simulink model "nav_flocking4"  (R2022b)
settings: Solver=FixedStepAuto  StartTime=0.0  StopTime=10.0  FixedStep=0.01  RelTol=1e-3
values from neighbouring files (symbols this model uses):
  a = 1    [main_flock3.m]    (also in main_flock4.m; params_flocking_ros.m)
  aR = diag([ar; ap; ay])    [main_flock3.m]    (also in main_flock4.m; main_sliding.m)
  Att1 = [2 -2 -15]    [main_flock3.m]    (also in main_flock4.m)
  Att2 = [2 -2 -15]    [main_flock3.m]    (also in main_flock4.m)
  Att3 = [2 -2 -15]    [main_flock3.m]    (also in main_flock4.m)
  Att4 = [2 -2 -15]    [main_flock4.m]
  b = 1    [main_flock3.m]    (also in main_flock4.m; params_flocking_ros.m)
  c = 1    [main_flock3.m]    (also in main_flock4.m; params_flocking_ros.m)
  c_gammap = 1.2    [main_flock3.m]    (also in main_flock4.m)
  c_gammav = 3.5    [main_flock3.m]    (also in main_flock4.m)
  d = 0.6    [main_flock3.m]    (also in main_flock4.m; params_flocking_ros.m)
  d_prime = 1    [main_flock3.m]    (also in main_flock4.m; params_flocking_ros.m)
  epsilon = 0.1    [main_flock3.m]    (also in main_flock4.m; params_flocking_ros.m)
  h = 0.2    [main_flock3.m]    (also in main_flock4.m; params_flocking_ros.m)
  K1 = diag([k111; k122; k133])    [main_flock3.m]    (also in main_flock4.m; main_sliding.m)
  K2 = diag([k211; k222; k233])    [main_flock3.m]    (also in main_flock4.m; main_sliding.m)
  Ki = diag([Ki1; Ki2; Ki3])    [main_flock3.m]    (also in main_flock4.m; main_sliding.m)
  lam = diag([lam1; lam2; lam3])    [main_flock3.m]    (also in main_flock4.m; main_sliding.m)
  R = 0.15    [main_flock3.m]    (also in main_flock4.m; params_flocking_ros.m)
  vxobs = 0    [main_flock3.m]    (also in main_flock4.m)
  vyobs = 0    [main_flock3.m]    (also in main_flock4.m)
  vzobs = 0    [main_flock3.m]    (also in main_flock4.m)
  X0_1 = [P01 dP01 om01]    [main_flock3.m]    (also in main_flock4.m; main_sliding.m = [P0 dP0 om0])
  X0_2 = [P02 dP02 om02]    [main_flock3.m]    (also in main_flock4.m)
  X0_3 = [P03 dP03 om03]    [main_flock3.m]    (also in main_flock4.m)
  X0_4 = [P04 dP04 om04]    [main_flock4.m]
  xmax = 2    [main_flock3.m]    (also in main_flock4.m)
  xmin = -2    [main_flock3.m]    (also in main_flock4.m)
  xobs = 0.75    [main_flock3.m]    (also in main_flock4.m)
  yobs = -0.25    [main_flock3.m]    (also in main_flock4.m)
  zobs = 1.7    [main_flock3.m]    (also in main_flock4.m)
undefined symbols (not defined in the file or in its folder): A_Euler
libraries: aerosimlib x4
(part 1 of 3)
settings Model: Creator=root  LastModifiedBy=jonatan_alvarez
settings SolverCC: AlgebraicLoopSolver=TrustRegion
settings DataIOCC: ReturnWorkspaceOutputs=off
settings DebuggingCC: UnconnectedInputMsg=warning  UnconnectedOutputMsg=warning  UnconnectedLineMsg=warning  SFMachineParentedDataDiag=warning  UnderSpecifiedDimensionMsg=warning  ArithmeticOperatorsInVariantConditions=warning
settings ModelReferenceCC: EnableRefExpFcnMdlSchedulingChecks=on
settings SFSimCC: CustomCodeUndefinedFunction=UseInterfaceOnly

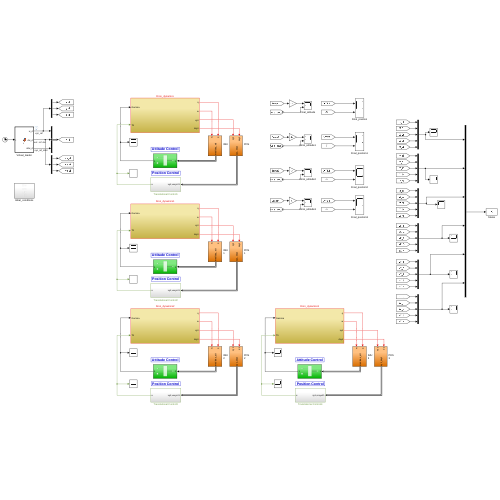
[thumbnail: Simulink's stored preview of the top-level diagram]
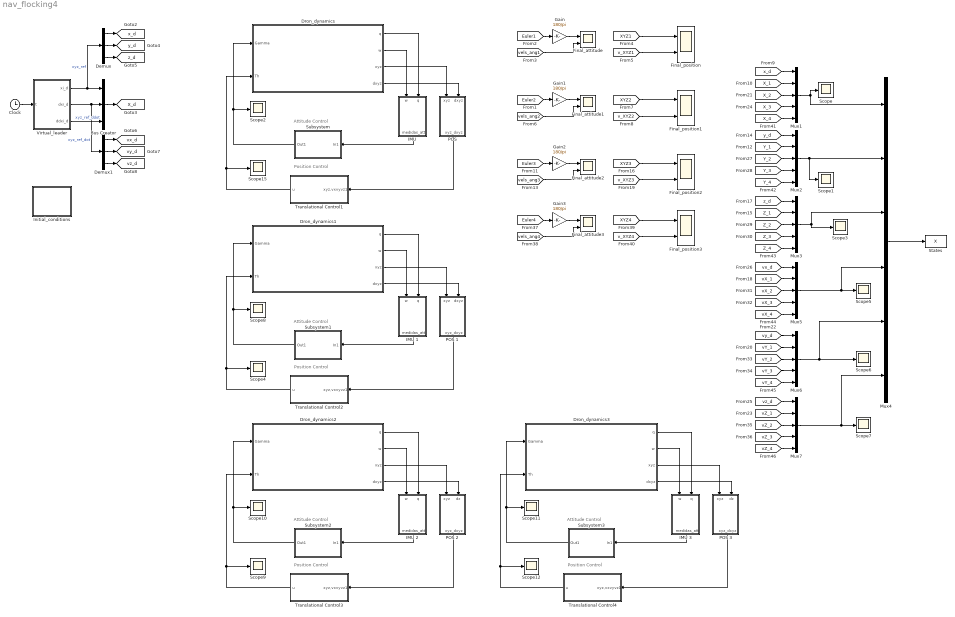
== system nav_flocking4 ==
  note: Position Control
  note: Attitude Control
  note: Position Control
  note: Attitude Control
  note: Position Control
  note: Attitude Control
  note: Position Control
  note: Attitude Control
  Bus Creator : BusCreator  Inputs=3
  Clock : Clock
  Demux : Demux  Outputs=3
  Demux1 : Demux  Outputs=3
  Dron_dynamics : Subsystem
  Dron_dynamics1 : Subsystem
  Dron_dynamics2 : Subsystem
  Dron_dynamics3 : Subsystem
  Final_attitude{,1..3} (4 alike) : Scope  NumInputPorts=2
  Final_position{,1..3} (4 alike) : Scope  NumInputPorts=2
  Gain{,1..3} (4 alike) : Gain  Gain=180/pi
  "IMU " : Subsystem
  IMU 1 : Subsystem
  IMU 2 : Subsystem
  IMU 3 : Subsystem
  Initial_conditions : Subsystem
  Mux{1..3,5..7} (6 alike) : Mux  Inputs=5
  Mux4 : Mux  Inputs=6
  "POS " : Subsystem
  POS 1 : Subsystem
  POS 2 : Subsystem
  POS 3 : Subsystem
  Scope{,1..12,15} (14 alike) : Scope
  States : ToWorkspace  VariableName=X  SampleTime=-1
  Subsystem : Subsystem
  Subsystem1 : Subsystem
  Subsystem2 : Subsystem
  Subsystem3 : Subsystem
  Translational Control1 : Subsystem
  Translational Control2 : Subsystem
  Translational Control3 : Subsystem
  Translational Control4 : Subsystem
  Virtual_leader : MATLAB Function  TreatAsAtomicUnit=on
  tag scope: X_d=global, vx_d=global, vy_d=global, vz_d=global, x_d=global, y_d=global, z_d=global
  wires:
  [vels_ang1] -> Final_attitude/2
  [v_XYZ1] -> Final_position/2
  Gain/1 -> Final_attitude/1
  [XYZ1] -> Final_position/1
  [Euler1] -> Gain/1
  Dron_dynamics/2(w) -> "IMU "/1(w)
  Dron_dynamics/4(dxyz) -> "POS "/2(dxyz)
  Bus Creator/1 -> [X_d]
  Virtual_leader/3(ddxi_d) -> Bus Creator/3  "xyz_ref_ddot"
  Dron_dynamics/1(q) -> "IMU "/2(q)
  Subsystem/1(Out1) -> Scope2/1, Dron_dynamics/1(Gamma)
  Dron_dynamics/3(xyz) -> "POS "/1(xyz)
  "POS "/1(xyz_dxyz) -> Translational Control1/1(xyz,vxvyvz1)
  Translational Control1/1(u) -> Scope15/1, Dron_dynamics/2(Th)
  "IMU "/1(medidas_att) -> Subsystem/1(In1)
  Virtual_leader/1(xi_d) -> Demux/1, Bus Creator/1  "xyz_ref"
  Demux/1 -> [x_d]
  Demux/2 -> [y_d]
  Demux/3 -> [z_d]
  [x_d] -> Mux1/1
  [X_1] -> Mux1/2
  Mux2/1 -> Scope1/1, Mux4/2
  [Y_1] -> Mux2/2
  [y_d] -> Mux2/1
  [z_d] -> Mux3/1
  [Z_1] -> Mux3/2
  Mux3/1 -> Mux4/3, Scope3/1
  Mux4/1 -> States/1
  Mux1/1 -> Scope/1, Mux4/1
  Demux1/3 -> [vz_d]
  Demux1/2 -> [vy_d]
  Demux1/1 -> [vx_d]
  Virtual_leader/2(dxi_d) -> Demux1/1, Bus Creator/2  "xyz_ref_dot"
  [vZ_1] -> Mux7/2
  [vz_d] -> Mux7/1
  [vy_d] -> Mux6/1
  [vY_1] -> Mux6/2
  [vX_1] -> Mux5/2
  [vx_d] -> Mux5/1
  Mux5/1 -> Mux4/4, Scope5/1
  Mux6/1 -> Mux4/5, Scope6/1
  Mux7/1 -> Mux4/6, Scope7/1
  Clock/1 -> Virtual_leader/1(t)
  Dron_dynamics1/2(w) -> IMU 1/1(w)
  Dron_dynamics1/4(dxyz) -> POS 1/2(dxyz)
  Dron_dynamics1/3(xyz) -> POS 1/1(xyz)
  POS 1/1(xyz_dxyz) -> Translational Control2/1(xyz,vxvyvz1)
  Dron_dynamics1/1(q) -> IMU 1/2(q)
  Translational Control2/1(u) -> Scope4/1, Dron_dynamics1/2(Th)
  IMU 1/1(medidas_att) -> Subsystem1/1(In1)
  Subsystem1/1(Out1) -> Scope8/1, Dron_dynamics1/1(Gamma)
  Dron_dynamics2/2(w) -> IMU 2/1(w)
  Dron_dynamics2/4(dxyz) -> POS 2/2(dz)
  Dron_dynamics2/3(xyz) -> POS 2/1(xyz)
  POS 2/1(xyz_dxyz) -> Translational Control3/1(xyz,vxvyvz1)
  Dron_dynamics2/1(q) -> IMU 2/2(q)
  Translational Control3/1(u) -> Scope9/1, Dron_dynamics2/2(Th)
  IMU 2/1(medidas_att) -> Subsystem2/1(In1)
  Subsystem2/1(Out1) -> Scope10/1, Dron_dynamics2/1(Gamma)
  [v_XYZ2] -> Final_position1/2
  [Euler2] -> Gain1/1
  Gain1/1 -> Final_attitude1/1
  [XYZ2] -> Final_position1/1
  [vels_ang2] -> Final_attitude1/2
  [v_XYZ3] -> Final_position2/2
  [Euler3] -> Gain2/1
  Gain2/1 -> Final_attitude2/1
  [XYZ3] -> Final_position2/1
  [vels_ang3] -> Final_attitude2/2
  [X_2] -> Mux1/3
  [X_3] -> Mux1/4
  [Y_2] -> Mux2/3
  [Y_3] -> Mux2/4
  [Z_2] -> Mux3/3
  [Z_3] -> Mux3/4
  [vX_2] -> Mux5/3
  [vX_3] -> Mux5/4
  [vY_2] -> Mux6/3
  [vY_3] -> Mux6/4
  [vZ_2] -> Mux7/3
  [vZ_3] -> Mux7/4
  Subsystem3/1(Out1) -> Dron_dynamics3/1(Gamma), Scope11/1
  IMU 3/1(medidas_att) -> Subsystem3/1(In1)
  Translational Control4/1(u) -> Dron_dynamics3/2(Th), Scope12/1
  Dron_dynamics3/1(q) -> IMU 3/2(q)
  POS 3/1(xyz_dxyz) -> Translational Control4/1(xyz,vxvyvz1)
  Dron_dynamics3/3(xyz) -> POS 3/1(xyz)
  Dron_dynamics3/4(dxyz) -> POS 3/2(dz)
  Dron_dynamics3/2(w) -> IMU 3/1(w)
  [vels_ang4] -> Final_attitude3/2
  [XYZ4] -> Final_position3/1
  Gain3/1 -> Final_attitude3/1
  [Euler4] -> Gain3/1
  [v_XYZ4] -> Final_position3/2
  [X_4] -> Mux1/5
  [Y_4] -> Mux2/5
  [Z_4] -> Mux3/5
  [vX_4] -> Mux5/5
  [vY_4] -> Mux6/5
  [vZ_4] -> Mux7/5

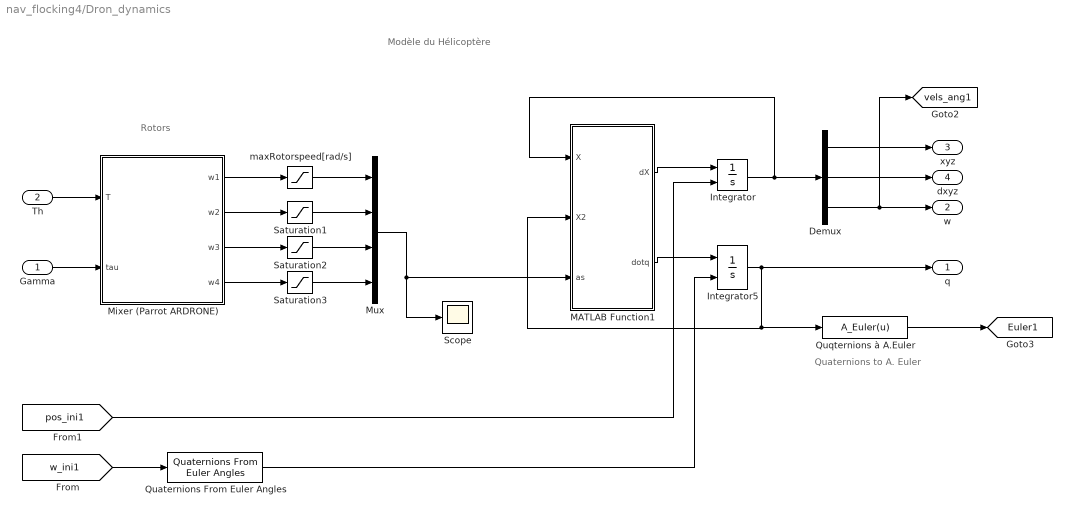
== system nav_flocking4/Dron_dynamics ==
  note: Modèle du Hélicoptère
  note: Rotors
  note: Quaternions to A. Euler
  Gamma : Inport
  Th : Inport  Port=2
  Demux : Demux  Outputs=3
  Integrator : Integrator  InitialConditionSource=external
  Integrator5 : Integrator  InitialConditionSource=external  InitialCondition=[1 0 0 0]
  MATLAB Function1 : MATLAB Function  TreatAsAtomicUnit=on
  Mixer (Parrot ARDRONE) : MATLAB Function  TreatAsAtomicUnit=on
  Mux : Mux
  Quaternions From Euler Angles : aerosimlib/Transformations/Quaternions From Euler Angles
  Quqternions à A.Euler : MATLABFcn  MATLABFcn=A_Euler(u)  OutputDimensions=3
  Saturation1 : Saturate  UpperLimit=1100  LowerLimit=5
  Saturation2 : Saturate  UpperLimit=1100  LowerLimit=5
  Saturation3 : Saturate  UpperLimit=1100  LowerLimit=5
  Scope : Scope
  maxRotorspeed[rad/s] : Saturate  UpperLimit=1100  LowerLimit=5
  q : Outport  VectorParamsAs1DForOutWhenUnconnected=off
  w : Outport  Port=2  VectorParamsAs1DForOutWhenUnconnected=off
  xyz : Outport  Port=3  VectorParamsAs1DForOutWhenUnconnected=off
  dxyz : Outport  Port=4  VectorParamsAs1DForOutWhenUnconnected=off
  tag scope: Euler1=global, vels_ang1=global
  wires:
  [w_ini1] -> Quaternions From Euler Angles/1
  Quqternions à A.Euler/1 -> [Euler1]
  Mixer (Parrot ARDRONE)/4(w4) -> Saturation3/1
  Saturation1/1 -> Mux/2
  Mixer (Parrot ARDRONE)/2(w2) -> Saturation1/1
  Mixer (Parrot ARDRONE)/1(w1) -> maxRotorspeed[rad/s]/1
  maxRotorspeed[rad/s]/1 -> Mux/1
  Saturation3/1 -> Mux/4
  Saturation2/1 -> Mux/3
  Mixer (Parrot ARDRONE)/3(w3) -> Saturation2/1
  Mux/1 -> Scope/1, MATLAB Function1/3(as)
  Integrator5/1 -> MATLAB Function1/2(X2), Quqternions à A.Euler/1, q/1
  MATLAB Function1/1(dX) -> Integrator/1
  MATLAB Function1/2(dotq) -> Integrator5/1
  Quaternions From Euler Angles/1 -> Integrator5/2
  Integrator/1 -> Demux/1, MATLAB Function1/1(X)
  Gamma/1 -> Mixer (Parrot ARDRONE)/2(tau)
  [pos_ini1] -> Integrator/2
  Demux/3 -> [vels_ang1], w/1
  Demux/1 -> xyz/1
  Demux/2 -> dxyz/1
  Th/1 -> Mixer (Parrot ARDRONE)/1(T)

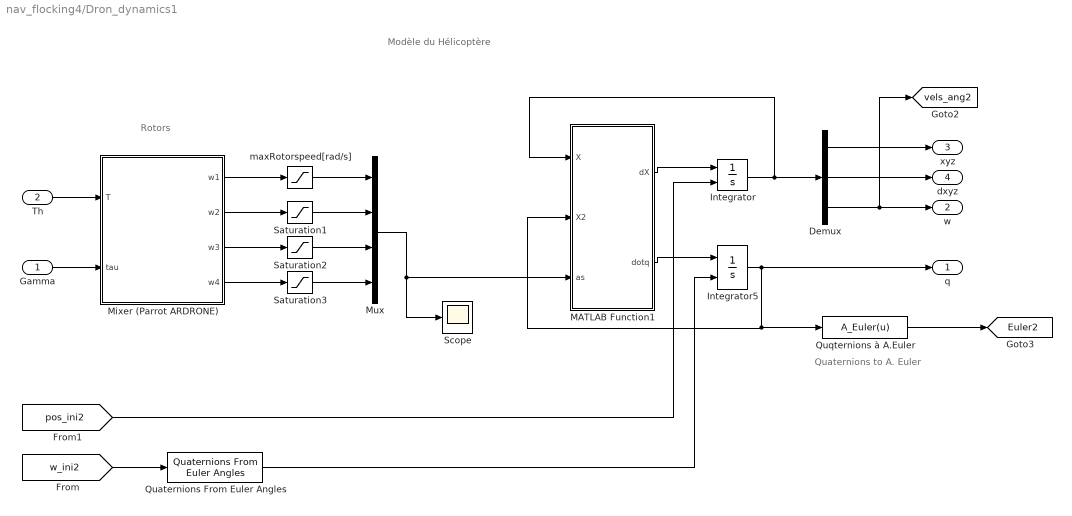
== system nav_flocking4/Dron_dynamics1 ==
  note: Modèle du Hélicoptère
  note: Rotors
  note: Quaternions to A. Euler
  Gamma : Inport
  Th : Inport  Port=2
  Demux : Demux  Outputs=3
  Integrator : Integrator  InitialConditionSource=external
  Integrator5 : Integrator  InitialConditionSource=external  InitialCondition=[1 0 0 0]
  MATLAB Function1 : MATLAB Function  TreatAsAtomicUnit=on
  Mixer (Parrot ARDRONE) : MATLAB Function  TreatAsAtomicUnit=on
  Mux : Mux
  Quaternions From Euler Angles : aerosimlib/Transformations/Quaternions From Euler Angles
  Quqternions à A.Euler : MATLABFcn  MATLABFcn=A_Euler(u)  OutputDimensions=3
  Saturation1 : Saturate  UpperLimit=1100  LowerLimit=5
  Saturation2 : Saturate  UpperLimit=1100  LowerLimit=5
  Saturation3 : Saturate  UpperLimit=1100  LowerLimit=5
  Scope : Scope
  maxRotorspeed[rad/s] : Saturate  UpperLimit=1100  LowerLimit=5
  q : Outport  VectorParamsAs1DForOutWhenUnconnected=off
  w : Outport  Port=2  VectorParamsAs1DForOutWhenUnconnected=off
  xyz : Outport  Port=3  VectorParamsAs1DForOutWhenUnconnected=off
  dxyz : Outport  Port=4  VectorParamsAs1DForOutWhenUnconnected=off
  tag scope: Euler2=global, vels_ang2=global
  wires:
  [w_ini2] -> Quaternions From Euler Angles/1
  Quqternions à A.Euler/1 -> [Euler2]
  Mixer (Parrot ARDRONE)/4(w4) -> Saturation3/1
  Saturation1/1 -> Mux/2
  Mixer (Parrot ARDRONE)/2(w2) -> Saturation1/1
  Mixer (Parrot ARDRONE)/1(w1) -> maxRotorspeed[rad/s]/1
  maxRotorspeed[rad/s]/1 -> Mux/1
  Saturation3/1 -> Mux/4
  Saturation2/1 -> Mux/3
  Mixer (Parrot ARDRONE)/3(w3) -> Saturation2/1
  Mux/1 -> Scope/1, MATLAB Function1/3(as)
  Integrator5/1 -> MATLAB Function1/2(X2), Quqternions à A.Euler/1, q/1
  MATLAB Function1/1(dX) -> Integrator/1
  MATLAB Function1/2(dotq) -> Integrator5/1
  Quaternions From Euler Angles/1 -> Integrator5/2
  Integrator/1 -> Demux/1, MATLAB Function1/1(X)
  Gamma/1 -> Mixer (Parrot ARDRONE)/2(tau)
  [pos_ini2] -> Integrator/2
  Demux/3 -> [vels_ang2], w/1
  Demux/1 -> xyz/1
  Demux/2 -> dxyz/1
  Th/1 -> Mixer (Parrot ARDRONE)/1(T)

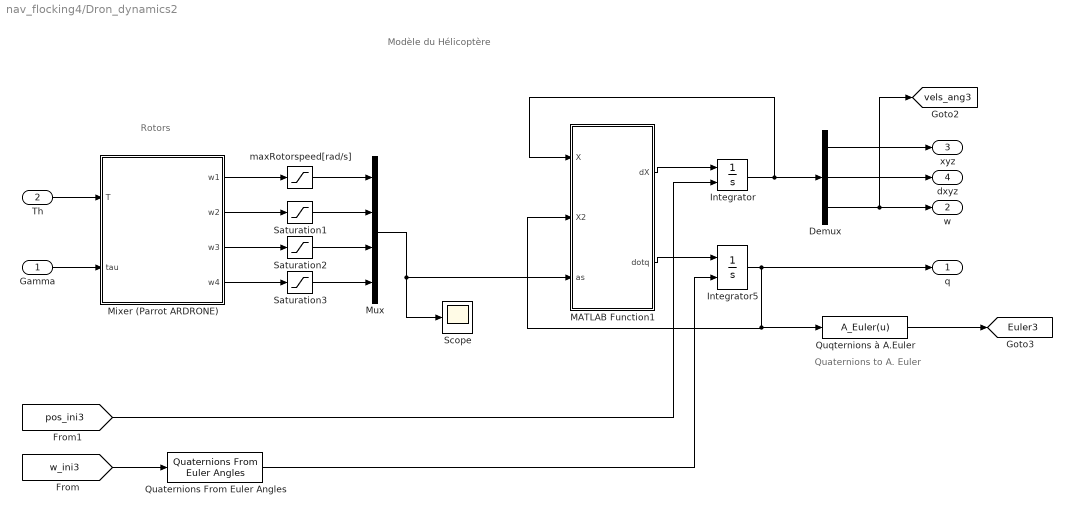
== system nav_flocking4/Dron_dynamics2 ==
  note: Modèle du Hélicoptère
  note: Rotors
  note: Quaternions to A. Euler
  Gamma : Inport
  Th : Inport  Port=2
  Demux : Demux  Outputs=3
  Integrator : Integrator  InitialConditionSource=external
  Integrator5 : Integrator  InitialConditionSource=external  InitialCondition=[1 0 0 0]
  MATLAB Function1 : MATLAB Function  TreatAsAtomicUnit=on
  Mixer (Parrot ARDRONE) : MATLAB Function  TreatAsAtomicUnit=on
  Mux : Mux
  Quaternions From Euler Angles : aerosimlib/Transformations/Quaternions From Euler Angles
  Quqternions à A.Euler : MATLABFcn  MATLABFcn=A_Euler(u)  OutputDimensions=3
  Saturation1 : Saturate  UpperLimit=1100  LowerLimit=5
  Saturation2 : Saturate  UpperLimit=1100  LowerLimit=5
  Saturation3 : Saturate  UpperLimit=1100  LowerLimit=5
  Scope : Scope
  maxRotorspeed[rad/s] : Saturate  UpperLimit=1100  LowerLimit=5
  q : Outport  VectorParamsAs1DForOutWhenUnconnected=off
  w : Outport  Port=2  VectorParamsAs1DForOutWhenUnconnected=off
  xyz : Outport  Port=3  VectorParamsAs1DForOutWhenUnconnected=off
  dxyz : Outport  Port=4  VectorParamsAs1DForOutWhenUnconnected=off
  tag scope: Euler3=global, vels_ang3=global
  wires:
  [w_ini3] -> Quaternions From Euler Angles/1
  Quqternions à A.Euler/1 -> [Euler3]
  Mixer (Parrot ARDRONE)/4(w4) -> Saturation3/1
  Saturation1/1 -> Mux/2
  Mixer (Parrot ARDRONE)/2(w2) -> Saturation1/1
  Mixer (Parrot ARDRONE)/1(w1) -> maxRotorspeed[rad/s]/1
  maxRotorspeed[rad/s]/1 -> Mux/1
  Saturation3/1 -> Mux/4
  Saturation2/1 -> Mux/3
  Mixer (Parrot ARDRONE)/3(w3) -> Saturation2/1
  Mux/1 -> Scope/1, MATLAB Function1/3(as)
  Integrator5/1 -> MATLAB Function1/2(X2), Quqternions à A.Euler/1, q/1
  MATLAB Function1/1(dX) -> Integrator/1
  MATLAB Function1/2(dotq) -> Integrator5/1
  Quaternions From Euler Angles/1 -> Integrator5/2
  Integrator/1 -> Demux/1, MATLAB Function1/1(X)
  Gamma/1 -> Mixer (Parrot ARDRONE)/2(tau)
  [pos_ini3] -> Integrator/2
  Demux/3 -> [vels_ang3], w/1
  Demux/1 -> xyz/1
  Demux/2 -> dxyz/1
  Th/1 -> Mixer (Parrot ARDRONE)/1(T)

== system nav_flocking4/Dron_dynamics3 ==
  note: Quaternions to A. Euler
  note: Rotors
  note: Modèle du Hélicoptère
  Gamma : Inport
  Th : Inport  Port=2
  Demux : Demux  Outputs=3
  Integrator : Integrator  InitialConditionSource=external
  Integrator5 : Integrator  InitialConditionSource=external  InitialCondition=[1 0 0 0]
  MATLAB Function1 : MATLAB Function  TreatAsAtomicUnit=on
  Mixer (Parrot ARDRONE) : MATLAB Function  TreatAsAtomicUnit=on
  Mux : Mux
  Quaternions From Euler Angles : aerosimlib/Transformations/Quaternions From Euler Angles
  Quqternions à A.Euler : MATLABFcn  MATLABFcn=A_Euler(u)  OutputDimensions=3
  Saturation1 : Saturate  UpperLimit=1100  LowerLimit=5
  Saturation2 : Saturate  UpperLimit=1100  LowerLimit=5
  Saturation3 : Saturate  UpperLimit=1100  LowerLimit=5
  Scope : Scope
  maxRotorspeed[rad/s] : Saturate  UpperLimit=1100  LowerLimit=5
  q : Outport  VectorParamsAs1DForOutWhenUnconnected=off
  w : Outport  Port=2  VectorParamsAs1DForOutWhenUnconnected=off
  xyz : Outport  Port=3  VectorParamsAs1DForOutWhenUnconnected=off
  dxyz : Outport  Port=4  VectorParamsAs1DForOutWhenUnconnected=off
  tag scope: Euler4=global, vels_ang4=global
  wires:
  Th/1 -> Mixer (Parrot ARDRONE)/1(T)
  Demux/2 -> dxyz/1
  Demux/1 -> xyz/1
  Demux/3 -> w/1, [vels_ang4]
  [pos_ini4] -> Integrator/2
  Gamma/1 -> Mixer (Parrot ARDRONE)/2(tau)
  Integrator/1 -> MATLAB Function1/1(X), Demux/1
  Quaternions From Euler Angles/1 -> Integrator5/2
  MATLAB Function1/2(dotq) -> Integrator5/1
  MATLAB Function1/1(dX) -> Integrator/1
  Integrator5/1 -> q/1, Quqternions à A.Euler/1, MATLAB Function1/2(X2)
  Mux/1 -> MATLAB Function1/3(as), Scope/1
  Mixer (Parrot ARDRONE)/3(w3) -> Saturation2/1
  Saturation2/1 -> Mux/3
  Saturation3/1 -> Mux/4
  maxRotorspeed[rad/s]/1 -> Mux/1
  Mixer (Parrot ARDRONE)/1(w1) -> maxRotorspeed[rad/s]/1
  Mixer (Parrot ARDRONE)/2(w2) -> Saturation1/1
  Saturation1/1 -> Mux/2
  Mixer (Parrot ARDRONE)/4(w4) -> Saturation3/1
  Quqternions à A.Euler/1 -> [Euler4]
  [w_ini4] -> Quaternions From Euler Angles/1

== system nav_flocking4/IMU  ==
  w : Inport
  q : Inport  Port=2
  Bus Creator : BusCreator  Inputs=4
  Display : Display
  Integrator : Integrator
  Scope : Scope
  q_e : Subsystem
  medidas_att : Outport  VectorParamsAs1DForOutWhenUnconnected=off
  wires:
  [q_d1] -> q_e/1(q1)
  q/1 -> Bus Creator/1, q_e/2(Q2)
  w/1 -> Bus Creator/3
  Integrator/1 -> Display/1, Bus Creator/4
  Bus Creator/1 -> medidas_att/1
  q_e/1(qxQ) -> Integrator/1, Scope/1, Bus Creator/2

== system nav_flocking4/IMU 1 ==
  w : Inport
  q : Inport  Port=2
  Bus Creator : BusCreator  Inputs=4
  Display : Display
  Integrator : Integrator
  Scope : Scope
  q_e : Subsystem
  medidas_att : Outport  VectorParamsAs1DForOutWhenUnconnected=off
  wires:
  [q_d2] -> q_e/1(q1)
  q/1 -> Bus Creator/1, q_e/2(Q2)
  w/1 -> Bus Creator/3
  Integrator/1 -> Display/1, Bus Creator/4
  Bus Creator/1 -> medidas_att/1
  q_e/1(qxQ) -> Integrator/1, Scope/1, Bus Creator/2

== system nav_flocking4/IMU 2 ==
  w : Inport
  q : Inport  Port=2
  Bus Creator : BusCreator  Inputs=4
  Display : Display
  Integrator : Integrator
  Scope : Scope
  q_e : Subsystem
  medidas_att : Outport  VectorParamsAs1DForOutWhenUnconnected=off
  wires:
  [q_d3] -> q_e/1(q1)
  q/1 -> Bus Creator/1, q_e/2(Q2)
  w/1 -> Bus Creator/3
  Integrator/1 -> Display/1, Bus Creator/4
  Bus Creator/1 -> medidas_att/1
  q_e/1(qxQ) -> Integrator/1, Scope/1, Bus Creator/2

== system nav_flocking4/IMU 3 ==
  w : Inport
  q : Inport  Port=2
  Bus Creator : BusCreator  Inputs=4
  Display : Display
  Integrator : Integrator
  Scope : Scope
  q_e : Subsystem
  medidas_att : Outport  VectorParamsAs1DForOutWhenUnconnected=off
  wires:
  q_e/1(qxQ) -> Bus Creator/2, Scope/1, Integrator/1
  Bus Creator/1 -> medidas_att/1
  Integrator/1 -> Bus Creator/4, Display/1
  w/1 -> Bus Creator/3
  q/1 -> q_e/2(Q2), Bus Creator/1
  [q_d4] -> q_e/1(q1)

== system nav_flocking4/Initial_conditions ==
  "phi, theta,psi Condition Initiale" : Constant  Value=[Att1]*pi/180
  "phi, theta,psi Condition Initiale1" : Constant  Value=X0_1
  "phi, theta,psi Condition Initiale2" : Constant  Value=[Att2]*pi/180
  "phi, theta,psi Condition Initiale3" : Constant  Value=X0_2
  "phi, theta,psi Condition Initiale4" : Constant  Value=[Att3]*pi/180
  "phi, theta,psi Condition Initiale5" : Constant  Value=X0_3
  "phi, theta,psi Condition Initiale6" : Constant  Value=[Att4]*pi/180
  "phi, theta,psi Condition Initiale7" : Constant  Value=X0_4
  tag scope: pos_ini1=global, pos_ini2=global, pos_ini3=global, pos_ini4=global, w_ini1=global, w_ini2=global, w_ini3=global, w_ini4=global
  wires:
  "phi, theta,psi Condition Initiale1"/1 -> [pos_ini1]
  "phi, theta,psi Condition Initiale"/1 -> [w_ini1]
  "phi, theta,psi Condition Initiale2"/1 -> [w_ini2]
  "phi, theta,psi Condition Initiale3"/1 -> [pos_ini2]
  "phi, theta,psi Condition Initiale4"/1 -> [w_ini3]
  "phi, theta,psi Condition Initiale5"/1 -> [pos_ini3]
  "phi, theta,psi Condition Initiale7"/1 -> [pos_ini4]
  "phi, theta,psi Condition Initiale6"/1 -> [w_ini4]

== system nav_flocking4/POS  ==
  xyz : Inport
  dxyz : Inport  Port=2
  Bus Creator : BusCreator  Inputs=2
  Demux : Demux  Outputs=3
  Demux1 : Demux  Outputs=3
  States : ToWorkspace  VariableName=X1  SampleTime=-1
  xyz_dxyz : Outport  VectorParamsAs1DForOutWhenUnconnected=off
  tag scope: XYZ1=global, X_1=global, Y_1=global, Z_1=global, states1=global, vX_1=global, vY_1=global, vZ_1=global, v_XYZ1=global
  wires:
  xyz/1 -> Bus Creator/1, States/1, Demux/1, [XYZ1]  "xyz"
  dxyz/1 -> Bus Creator/2, Demux1/1, [v_XYZ1]  "xyz_dot"
  Demux/1 -> [X_1]
  Demux/2 -> [Y_1]
  Demux/3 -> [Z_1]
  Demux1/3 -> [vZ_1]
  Demux1/2 -> [vY_1]
  Demux1/1 -> [vX_1]
  Bus Creator/1 -> [states1], xyz_dxyz/1

== system nav_flocking4/POS 1 ==
  xyz : Inport
  dxyz : Inport  Port=2
  Bus Creator : BusCreator  Inputs=2
  Demux : Demux  Outputs=3
  Demux1 : Demux  Outputs=3
  States : ToWorkspace  VariableName=X2  SampleTime=-1
  xyz_dxyz : Outport  VectorParamsAs1DForOutWhenUnconnected=off
  tag scope: XYZ2=global, X_2=global, Y_2=global, Z_2=global, states2=global, vX_2=global, vY_2=global, vZ_2=global, v_XYZ2=global
  wires:
  xyz/1 -> Bus Creator/1, States/1, Demux/1, [XYZ2]  "xyz"
  dxyz/1 -> Bus Creator/2, Demux1/1, [v_XYZ2]  "xyz_dot"
  Demux/1 -> [X_2]
  Demux/2 -> [Y_2]
  Demux/3 -> [Z_2]
  Bus Creator/1 -> [states2], xyz_dxyz/1
  Demux1/3 -> [vZ_2]
  Demux1/2 -> [vY_2]
  Demux1/1 -> [vX_2]

== system nav_flocking4/POS 2 ==
  xyz : Inport
  dz : Inport  Port=2
  Bus Creator : BusCreator  Inputs=2
  Demux : Demux  Outputs=3
  Demux1 : Demux  Outputs=3
  States : ToWorkspace  VariableName=X3  SampleTime=-1
  xyz_dxyz : Outport  VectorParamsAs1DForOutWhenUnconnected=off
  tag scope: XYZ3=global, X_3=global, Y_3=global, Z_3=global, states3=global, vX_3=global, vY_3=global, vZ_3=global, v_XYZ3=global
  wires:
  xyz/1 -> Bus Creator/1, States/1, Demux/1, [XYZ3]  "xyz"
  dz/1 -> Bus Creator/2, Demux1/1, [v_XYZ3]  "xyz_dot"
  Demux/1 -> [X_3]
  Demux/2 -> [Y_3]
  Demux/3 -> [Z_3]
  Bus Creator/1 -> [states3], xyz_dxyz/1
  Demux1/3 -> [vZ_3]
  Demux1/2 -> [vY_3]
  Demux1/1 -> [vX_3]

== system nav_flocking4/POS 3 ==
  xyz : Inport
  dz : Inport  Port=2
  Bus Creator : BusCreator  Inputs=2
  Demux : Demux  Outputs=3
  Demux1 : Demux  Outputs=3
  States : ToWorkspace  VariableName=X4  SampleTime=-1
  xyz_dxyz : Outport  VectorParamsAs1DForOutWhenUnconnected=off
  tag scope: XYZ4=global, X_4=global, Y_4=global, Z_4=global, states4=global, vX_4=global, vY_4=global, vZ_4=global, v_XYZ4=global
  wires:
  Demux1/1 -> [vX_4]
  Demux1/2 -> [vY_4]
  Demux1/3 -> [vZ_4]
  Bus Creator/1 -> xyz_dxyz/1, [states4]
  Demux/3 -> [Z_4]
  Demux/2 -> [Y_4]
  Demux/1 -> [X_4]
  dz/1 -> [v_XYZ4], Demux1/1, Bus Creator/2  "xyz_dot"
  xyz/1 -> [XYZ4], Demux/1, States/1, Bus Creator/1  "xyz"

== system nav_flocking4/Subsystem ==
  In1 : Inport
  Scope : Scope
  Sliding mode (quaternions) : MATLAB Function  Description=Integral quaternion Sliding mode control  TreatAsAtomicUnit=on
  Out1 : Outport  VectorParamsAs1DForOutWhenUnconnected=off
  wires:
  In1/1 -> Sliding mode (quaternions)/1(qwe)
  Sliding mode (quaternions)/1(Gamma) -> Out1/1
  Sliding mode (quaternions)/2(s) -> Scope/1

== system nav_flocking4/Subsystem1 ==
  In1 : Inport
  Scope : Scope
  Sliding mode (quaternions) : MATLAB Function  Description=Integral quaternion Sliding mode control  TreatAsAtomicUnit=on
  Out1 : Outport  VectorParamsAs1DForOutWhenUnconnected=off
  wires:
  In1/1 -> Sliding mode (quaternions)/1(qwe)
  Sliding mode (quaternions)/1(Gamma) -> Out1/1
  Sliding mode (quaternions)/2(s) -> Scope/1

== system nav_flocking4/Subsystem2 ==
  In1 : Inport
  Scope : Scope
  Sliding mode (quaternions) : MATLAB Function  Description=Integral quaternion Sliding mode control  TreatAsAtomicUnit=on
  Out1 : Outport  VectorParamsAs1DForOutWhenUnconnected=off
  wires:
  In1/1 -> Sliding mode (quaternions)/1(qwe)
  Sliding mode (quaternions)/1(Gamma) -> Out1/1
  Sliding mode (quaternions)/2(s) -> Scope/1

== system nav_flocking4/Subsystem3 ==
  In1 : Inport
  Scope : Scope
  Sliding mode (quaternions) : MATLAB Function  Description=Integral quaternion Sliding mode control  TreatAsAtomicUnit=on
  Out1 : Outport  VectorParamsAs1DForOutWhenUnconnected=off
  wires:
  Sliding mode (quaternions)/2(s) -> Scope/1
  Sliding mode (quaternions)/1(Gamma) -> Out1/1
  In1/1 -> Sliding mode (quaternions)/1(qwe)

== system nav_flocking4/Translational Control1 ==
  xyz,vxvyvz1 : Inport
  Flocking1 : Subsystem
  Scope2 : Scope
  Scope3 : Scope
  to_desired_angles : MATLAB Function  TreatAsAtomicUnit=on
  u : Outport  VectorParamsAs1DForOutWhenUnconnected=off
  tag scope: q_d1=global, u_1=global
  wires:
  to_desired_angles/2(Uz) -> u/1
  to_desired_angles/1(cq_d) -> Scope2/1, [q_d1]
  [X_d] -> Flocking1/1(ref)
  xyz,vxvyvz1/1 -> Flocking1/2(state)
  Flocking1/1(U_i) -> [u_1], Scope3/1, to_desired_angles/1(Gamma)
  [states2] -> Flocking1/3(statej)
  [states3] -> Flocking1/4(statek)
  [states4] -> Flocking1/5(statek1)

== system nav_flocking4/Translational Control2 ==
  xyz,vxvyvz1 : Inport
  Flocking1 : Subsystem
  Scope2 : Scope
  Scope3 : Scope
  to_desired_angles : MATLAB Function  TreatAsAtomicUnit=on
  u : Outport  VectorParamsAs1DForOutWhenUnconnected=off
  tag scope: q_d2=global, u_2=global
  wires:
  to_desired_angles/2(Uz) -> u/1
  to_desired_angles/1(cq_d) -> Scope2/1, [q_d2]
  [X_d] -> Flocking1/1(ref)
  xyz,vxvyvz1/1 -> Flocking1/2(state)
  Flocking1/1(U_i) -> [u_2], Scope3/1, to_desired_angles/1(Gamma)
  [states1] -> Flocking1/3(statej)
  [states3] -> Flocking1/4(statek)
  [states4] -> Flocking1/5(statek1)

== system nav_flocking4/Translational Control3 ==
  xyz,vxvyvz1 : Inport
  Flocking1 : Subsystem
  Scope2 : Scope
  Scope3 : Scope
  to_desired_angles : MATLAB Function  TreatAsAtomicUnit=on
  u : Outport  VectorParamsAs1DForOutWhenUnconnected=off
  tag scope: q_d3=global, u_3=global
  wires:
  to_desired_angles/2(Uz) -> u/1
  to_desired_angles/1(cq_d) -> Scope2/1, [q_d3]
  [X_d] -> Flocking1/1(ref)
  xyz,vxvyvz1/1 -> Flocking1/2(state)
  Flocking1/1(U_i) -> [u_3], Scope3/1, to_desired_angles/1(Gamma)
  [states1] -> Flocking1/3(statej)
  [states2] -> Flocking1/4(statek)
  [states4] -> Flocking1/5(statek1)

== system nav_flocking4/Translational Control4 ==
  xyz,vxvyvz1 : Inport
  Flocking1 : Subsystem
  Scope2 : Scope
  Scope3 : Scope
  to_desired_angles : MATLAB Function  TreatAsAtomicUnit=on
  u : Outport  VectorParamsAs1DForOutWhenUnconnected=off
  tag scope: q_d4=global, u_4=global
  wires:
  [states2] -> Flocking1/4(statek)
  [states1] -> Flocking1/3(statej)
  Flocking1/1(U_i) -> to_desired_angles/1(Gamma), Scope3/1, [u_4]
  xyz,vxvyvz1/1 -> Flocking1/2(state)
  [X_d] -> Flocking1/1(ref)
  to_desired_angles/1(cq_d) -> [q_d4], Scope2/1
  to_desired_angles/2(Uz) -> u/1
  [states3] -> Flocking1/5(statek1)

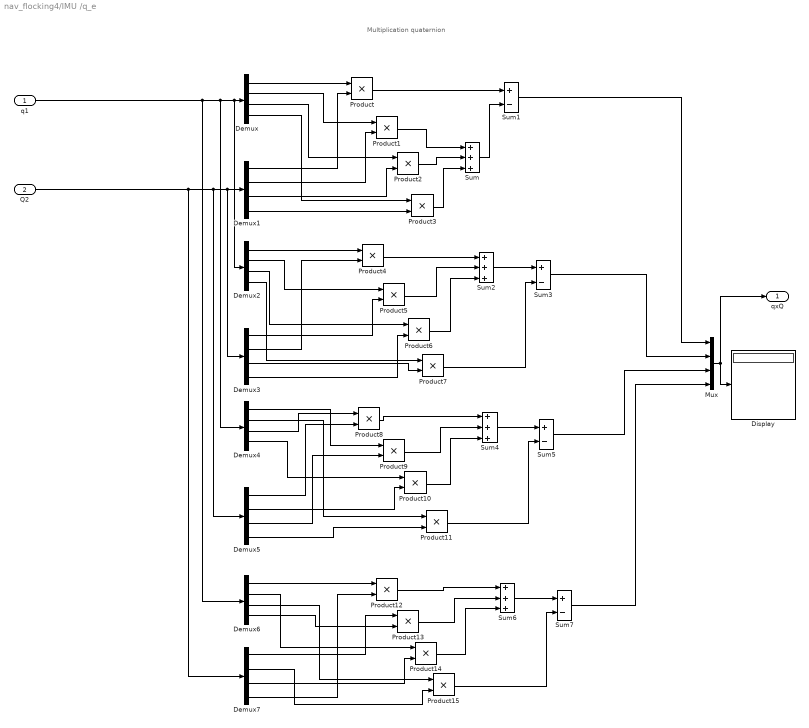
== system nav_flocking4/IMU /q_e ==
  note: Multiplication quaternion
  q1 : Inport
  Q2 : Inport  Port=2
  Demux{,1..7} (8 alike) : Demux
  Display : Display
  Mux : Mux
  Product{,1..15} (16 alike) : Product  RndMeth=Zero
  Sum{,2,4,6} (4 alike) : Sum  Inputs=+++
  Sum{1,3,5,7} (4 alike) : Sum  Inputs=+-
  qxQ : Outport  VectorParamsAs1DForOutWhenUnconnected=off
  wires:
  q1/1 -> Demux/1, Demux2/1, Demux4/1, Demux6/1
  Q2/1 -> Demux1/1, Demux3/1, Demux5/1, Demux7/1
  Demux/1 -> Product/1
  Demux1/1 -> Product/2
  Demux/2 -> Product1/1
  Demux1/2 -> Product1/2
  Demux/3 -> Product2/1
  Demux1/3 -> Product2/2
  Demux/4 -> Product3/1
  Demux1/4 -> Product3/2
  Product1/1 -> Sum/1
  Product2/1 -> Sum/2
  Product3/1 -> Sum/3
  Sum/1 -> Sum1/2
  Product/1 -> Sum1/1
  Demux2/1 -> Product4/1
  Demux3/2 -> Product4/2
  Demux2/2 -> Product5/1
  Demux3/1 -> Product5/2
  Demux2/3 -> Product6/1
  Demux3/4 -> Product6/2
  Demux2/4 -> Product7/1
  Demux3/3 -> Product7/2
  Product4/1 -> Sum2/1
  Product5/1 -> Sum2/2
  Product6/1 -> Sum2/3
  Sum2/1 -> Sum3/1
  Product7/1 -> Sum3/2
  Demux4/3 -> Product8/1
  Demux5/1 -> Product8/2
  Demux4/1 -> Product9/1
  Demux5/3 -> Product9/2
  Demux4/4 -> Product10/1
  Demux5/2 -> Product10/2
  Demux5/4 -> Product11/2
  Demux4/2 -> Product11/1
  Sum4/1 -> Sum5/1
  Product11/1 -> Sum5/2
  Product8/1 -> Sum4/1
  Product9/1 -> Sum4/2
  Product10/1 -> Sum4/3
  Demux6/1 -> Product12/1
  Demux7/1 -> Product13/1
  Demux6/2 -> Product14/1
  Demux7/4 -> Product12/2
  Demux6/4 -> Product13/2
  Demux7/3 -> Product14/2
  Demux6/3 -> Product15/1
  Demux7/2 -> Product15/2
  Sum6/1 -> Sum7/1
  Product15/1 -> Sum7/2
  Product12/1 -> Sum6/1
  Product13/1 -> Sum6/2
  Product14/1 -> Sum6/3
  Sum1/1 -> Mux/1
  Sum3/1 -> Mux/2
  Sum5/1 -> Mux/3
  Sum7/1 -> Mux/4
  Mux/1 -> Display/1, qxQ/1

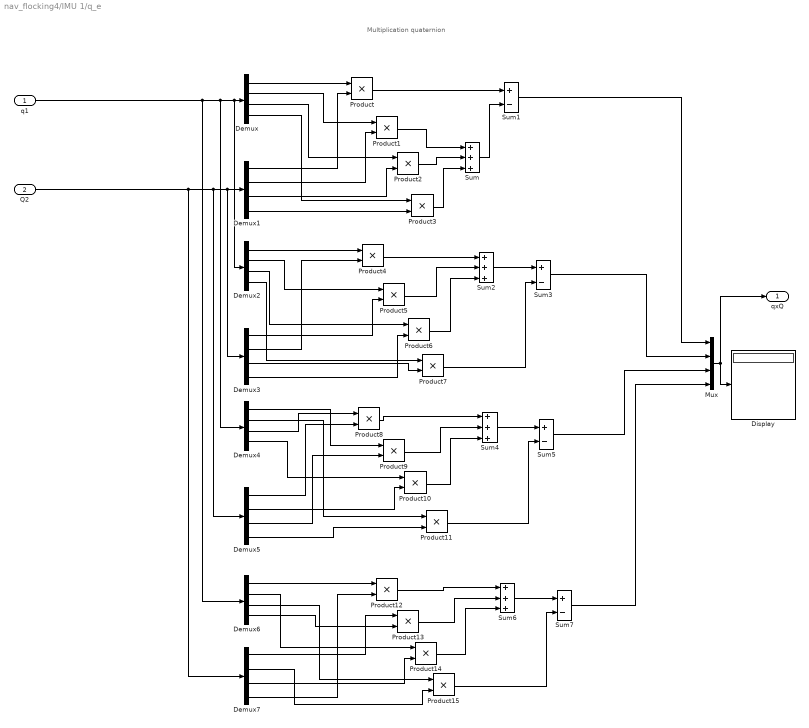
== system nav_flocking4/IMU 1/q_e ==
  note: Multiplication quaternion
  q1 : Inport
  Q2 : Inport  Port=2
  Demux{,1..7} (8 alike) : Demux
  Display : Display
  Mux : Mux
  Product{,1..15} (16 alike) : Product  RndMeth=Zero
  Sum{,2,4,6} (4 alike) : Sum  Inputs=+++
  Sum{1,3,5,7} (4 alike) : Sum  Inputs=+-
  qxQ : Outport  VectorParamsAs1DForOutWhenUnconnected=off
  wires:
  q1/1 -> Demux/1, Demux2/1, Demux4/1, Demux6/1
  Q2/1 -> Demux1/1, Demux3/1, Demux5/1, Demux7/1
  Demux/1 -> Product/1
  Demux1/1 -> Product/2
  Demux/2 -> Product1/1
  Demux1/2 -> Product1/2
  Demux/3 -> Product2/1
  Demux1/3 -> Product2/2
  Demux/4 -> Product3/1
  Demux1/4 -> Product3/2
  Product1/1 -> Sum/1
  Product2/1 -> Sum/2
  Product3/1 -> Sum/3
  Sum/1 -> Sum1/2
  Product/1 -> Sum1/1
  Demux2/1 -> Product4/1
  Demux3/2 -> Product4/2
  Demux2/2 -> Product5/1
  Demux3/1 -> Product5/2
  Demux2/3 -> Product6/1
  Demux3/4 -> Product6/2
  Demux2/4 -> Product7/1
  Demux3/3 -> Product7/2
  Product4/1 -> Sum2/1
  Product5/1 -> Sum2/2
  Product6/1 -> Sum2/3
  Sum2/1 -> Sum3/1
  Product7/1 -> Sum3/2
  Demux4/3 -> Product8/1
  Demux5/1 -> Product8/2
  Demux4/1 -> Product9/1
  Demux5/3 -> Product9/2
  Demux4/4 -> Product10/1
  Demux5/2 -> Product10/2
  Demux5/4 -> Product11/2
  Demux4/2 -> Product11/1
  Sum4/1 -> Sum5/1
  Product11/1 -> Sum5/2
  Product8/1 -> Sum4/1
  Product9/1 -> Sum4/2
  Product10/1 -> Sum4/3
  Demux6/1 -> Product12/1
  Demux7/1 -> Product13/1
  Demux6/2 -> Product14/1
  Demux7/4 -> Product12/2
  Demux6/4 -> Product13/2
  Demux7/3 -> Product14/2
  Demux6/3 -> Product15/1
  Demux7/2 -> Product15/2
  Sum6/1 -> Sum7/1
  Product15/1 -> Sum7/2
  Product12/1 -> Sum6/1
  Product13/1 -> Sum6/2
  Product14/1 -> Sum6/3
  Sum1/1 -> Mux/1
  Sum3/1 -> Mux/2
  Sum5/1 -> Mux/3
  Sum7/1 -> Mux/4
  Mux/1 -> Display/1, qxQ/1

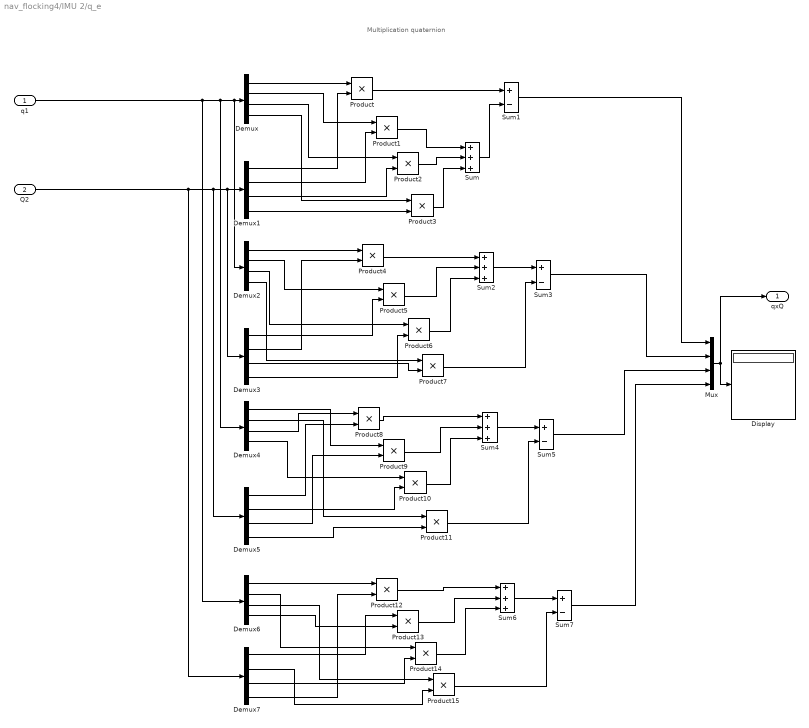
== system nav_flocking4/IMU 2/q_e ==
  note: Multiplication quaternion
  q1 : Inport
  Q2 : Inport  Port=2
  Demux{,1..7} (8 alike) : Demux
  Display : Display
  Mux : Mux
  Product{,1..15} (16 alike) : Product  RndMeth=Zero
  Sum{,2,4,6} (4 alike) : Sum  Inputs=+++
  Sum{1,3,5,7} (4 alike) : Sum  Inputs=+-
  qxQ : Outport  VectorParamsAs1DForOutWhenUnconnected=off
  wires:
  q1/1 -> Demux/1, Demux2/1, Demux4/1, Demux6/1
  Q2/1 -> Demux1/1, Demux3/1, Demux5/1, Demux7/1
  Demux/1 -> Product/1
  Demux1/1 -> Product/2
  Demux/2 -> Product1/1
  Demux1/2 -> Product1/2
  Demux/3 -> Product2/1
  Demux1/3 -> Product2/2
  Demux/4 -> Product3/1
  Demux1/4 -> Product3/2
  Product1/1 -> Sum/1
  Product2/1 -> Sum/2
  Product3/1 -> Sum/3
  Sum/1 -> Sum1/2
  Product/1 -> Sum1/1
  Demux2/1 -> Product4/1
  Demux3/2 -> Product4/2
  Demux2/2 -> Product5/1
  Demux3/1 -> Product5/2
  Demux2/3 -> Product6/1
  Demux3/4 -> Product6/2
  Demux2/4 -> Product7/1
  Demux3/3 -> Product7/2
  Product4/1 -> Sum2/1
  Product5/1 -> Sum2/2
  Product6/1 -> Sum2/3
  Sum2/1 -> Sum3/1
  Product7/1 -> Sum3/2
  Demux4/3 -> Product8/1
  Demux5/1 -> Product8/2
  Demux4/1 -> Product9/1
  Demux5/3 -> Product9/2
  Demux4/4 -> Product10/1
  Demux5/2 -> Product10/2
  Demux5/4 -> Product11/2
  Demux4/2 -> Product11/1
  Sum4/1 -> Sum5/1
  Product11/1 -> Sum5/2
  Product8/1 -> Sum4/1
  Product9/1 -> Sum4/2
  Product10/1 -> Sum4/3
  Demux6/1 -> Product12/1
  Demux7/1 -> Product13/1
  Demux6/2 -> Product14/1
  Demux7/4 -> Product12/2
  Demux6/4 -> Product13/2
  Demux7/3 -> Product14/2
  Demux6/3 -> Product15/1
  Demux7/2 -> Product15/2
  Sum6/1 -> Sum7/1
  Product15/1 -> Sum7/2
  Product12/1 -> Sum6/1
  Product13/1 -> Sum6/2
  Product14/1 -> Sum6/3
  Sum1/1 -> Mux/1
  Sum3/1 -> Mux/2
  Sum5/1 -> Mux/3
  Sum7/1 -> Mux/4
  Mux/1 -> Display/1, qxQ/1

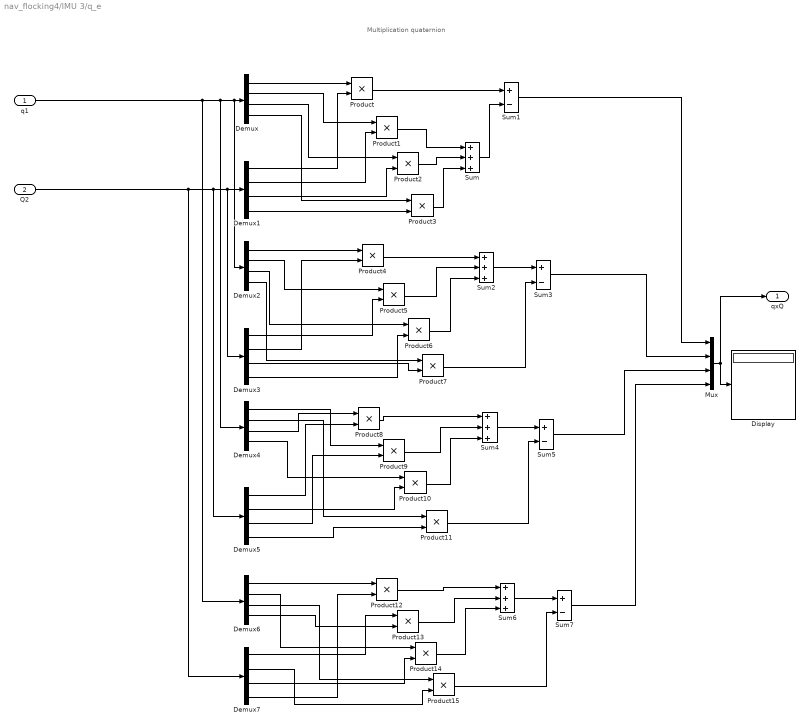
== system nav_flocking4/IMU 3/q_e ==
  note: Multiplication quaternion
  q1 : Inport
  Q2 : Inport  Port=2
  Demux{,1..7} (8 alike) : Demux
  Display : Display
  Mux : Mux
  Product{,1..15} (16 alike) : Product  RndMeth=Zero
  Sum{,2,4,6} (4 alike) : Sum  Inputs=+++
  Sum{1,3,5,7} (4 alike) : Sum  Inputs=+-
  qxQ : Outport  VectorParamsAs1DForOutWhenUnconnected=off
  wires:
  Mux/1 -> qxQ/1, Display/1
  Sum7/1 -> Mux/4
  Sum5/1 -> Mux/3
  Sum3/1 -> Mux/2
  Sum1/1 -> Mux/1
  Product14/1 -> Sum6/3
  Product13/1 -> Sum6/2
  Product12/1 -> Sum6/1
  Product15/1 -> Sum7/2
  Sum6/1 -> Sum7/1
  Demux7/2 -> Product15/2
  Demux6/3 -> Product15/1
  Demux7/3 -> Product14/2
  Demux6/4 -> Product13/2
  Demux7/4 -> Product12/2
  Demux6/2 -> Product14/1
  Demux7/1 -> Product13/1
  Demux6/1 -> Product12/1
  Product10/1 -> Sum4/3
  Product9/1 -> Sum4/2
  Product8/1 -> Sum4/1
  Product11/1 -> Sum5/2
  Sum4/1 -> Sum5/1
  Demux4/2 -> Product11/1
  Demux5/4 -> Product11/2
  Demux5/2 -> Product10/2
  Demux4/4 -> Product10/1
  Demux5/3 -> Product9/2
  Demux4/1 -> Product9/1
  Demux5/1 -> Product8/2
  Demux4/3 -> Product8/1
  Product7/1 -> Sum3/2
  Sum2/1 -> Sum3/1
  Product6/1 -> Sum2/3
  Product5/1 -> Sum2/2
  Product4/1 -> Sum2/1
  Demux3/3 -> Product7/2
  Demux2/4 -> Product7/1
  Demux3/4 -> Product6/2
  Demux2/3 -> Product6/1
  Demux3/1 -> Product5/2
  Demux2/2 -> Product5/1
  Demux3/2 -> Product4/2
  Demux2/1 -> Product4/1
  Product/1 -> Sum1/1
  Sum/1 -> Sum1/2
  Product3/1 -> Sum/3
  Product2/1 -> Sum/2
  Product1/1 -> Sum/1
  Demux1/4 -> Product3/2
  Demux/4 -> Product3/1
  Demux1/3 -> Product2/2
  Demux/3 -> Product2/1
  Demux1/2 -> Product1/2
  Demux/2 -> Product1/1
  Demux1/1 -> Product/2
  Demux/1 -> Product/1
  Q2/1 -> Demux7/1, Demux5/1, Demux3/1, Demux1/1
  q1/1 -> Demux6/1, Demux4/1, Demux2/1, Demux/1

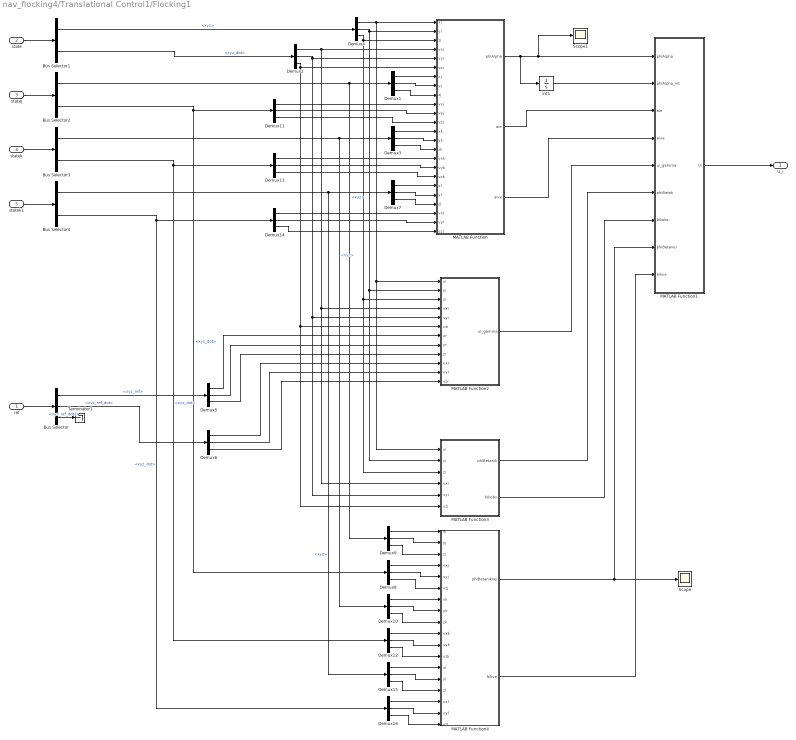
== system nav_flocking4/Translational Control1/Flocking1 ==
  ref : Inport
  state : Inport  Port=2
  statej : Inport  Port=3
  statek : Inport  Port=4
  statek1 : Inport  Port=5
  Bus Selector : BusSelector  OutputSignals=xyz_ref,xyz_ref_dot,xyz_ref_ddot
  Bus Selector{1..4} (4 alike) : BusSelector  OutputSignals=xyz,xyz_dot
  Demux{1..16} (16 alike) : Demux  Outputs=3
  MATLAB Function : MATLAB Function  TreatAsAtomicUnit=on
  MATLAB Function1 : MATLAB Function  TreatAsAtomicUnit=on
  MATLAB Function2 : MATLAB Function  TreatAsAtomicUnit=on
  MATLAB Function3 : MATLAB Function  TreatAsAtomicUnit=on
  MATLAB Function4 : MATLAB Function  TreatAsAtomicUnit=on
  Scope : Scope
  Scope1 : Scope
  Terminator1 : Terminator
  int1 : Integrator
  U_i : Outport  VectorParamsAs1DForOutWhenUnconnected=off
  wires:
  ref/1 -> Bus Selector/1
  state/1 -> Bus Selector1/1
  Bus Selector/2 -> Demux6/1  "<xyz_ref_dot>"
  Bus Selector/1 -> Demux5/1  "<xyz_ref>"
  Bus Selector1/1 -> Demux4/1  "<xyz>"
  Demux6/1 -> MATLAB Function2/10(vxr)
  Demux6/2 -> MATLAB Function2/11(vyr)
  statej/1 -> Bus Selector2/1
  Bus Selector2/1 -> Demux9/1, Demux1/1  "<xyz>"
  Demux4/1 -> MATLAB Function3/1(xi), MATLAB Function2/1(xi), MATLAB Function/1(xi)
  Demux4/2 -> MATLAB Function3/2(yi), MATLAB Function2/2(yi), MATLAB Function/2(yi)
  Demux1/1 -> MATLAB Function/7(xj)
  Demux1/2 -> MATLAB Function/8(yj)
  Bus Selector2/2 -> Demux8/1, Demux11/1  "<xyz_dot>"
  int1/1 -> MATLAB Function1/2(phiAlpha_int)
  MATLAB Function2/1(ui_gamma) -> MATLAB Function1/5(ui_gamma)
  statek/1 -> Bus Selector3/1
  Bus Selector3/2 -> Demux12/1, Demux13/1  "<xyz_dot>"
  Demux3/1 -> MATLAB Function/13(xk)
  Demux3/2 -> MATLAB Function/14(yk)
  Bus Selector3/1 -> Demux10/1, Demux3/1  "<xyz>"
  Demux9/1 -> MATLAB Function4/1(xj)
  Demux9/2 -> MATLAB Function4/2(yj)
  Demux10/1 -> MATLAB Function4/7(xk)
  Demux10/2 -> MATLAB Function4/8(yk)
  MATLAB Function/1(phiAlpha) -> int1/1, Scope1/1, MATLAB Function1/1(phiAlpha)
  Demux5/1 -> MATLAB Function2/7(xr)
  Demux5/2 -> MATLAB Function2/8(yr)
  Bus Selector1/2 -> Demux2/1  "<xyz_dot>"
  Demux4/3 -> MATLAB Function3/3(zi), MATLAB Function2/3(zi), MATLAB Function/3(zi)
  Demux3/3 -> MATLAB Function/15(zk)
  Demux5/3 -> MATLAB Function2/9(zr)
  Demux6/3 -> MATLAB Function2/12(vzr)
  MATLAB Function1/1(Ui) -> U_i/1
  Demux2/1 -> MATLAB Function2/4(vxi), MATLAB Function3/4(vxi), MATLAB Function/4(vxi)
  Demux2/2 -> MATLAB Function3/5(vyi), MATLAB Function2/5(vyi), MATLAB Function/5(vyi)
  Demux2/3 -> MATLAB Function3/6(vzi), MATLAB Function2/6(vzi), MATLAB Function/6(vzi)
  Demux1/3 -> MATLAB Function/9(zj)
  Demux11/1 -> MATLAB Function/10(vxj)
  Demux11/2 -> MATLAB Function/11(vyj)
  Demux11/3 -> MATLAB Function/12(vzj)
  Demux13/1 -> MATLAB Function/16(vxk)
  Demux13/2 -> MATLAB Function/17(vyk)
  Demux13/3 -> MATLAB Function/18(vzk)
  MATLAB Function/3(aive) -> MATLAB Function1/4(aive)
  Demux9/3 -> MATLAB Function4/3(zj)
  Demux10/3 -> MATLAB Function4/9(zk)
  MATLAB Function4/1(phiBetaniknei) -> Scope/1, MATLAB Function1/8(phiBetanei)
  Bus Selector/3 -> Terminator1/1  "<xyz_ref_ddot>"
  Demux8/1 -> MATLAB Function4/4(vxj)
  Demux8/2 -> MATLAB Function4/5(vyj)
  Demux8/3 -> MATLAB Function4/6(vzj)
  Demux12/1 -> MATLAB Function4/10(vxk)
  Demux12/2 -> MATLAB Function4/11(vyk)
  Demux12/3 -> MATLAB Function4/12(vzk)
  MATLAB Function4/2(bikve) -> MATLAB Function1/9(bikve)
  MATLAB Function3/1(phiBetanik) -> MATLAB Function1/6(phiBetak)
  MATLAB Function3/2(bikobs) -> MATLAB Function1/7(bikobs)
  MATLAB Function/2(aie) -> MATLAB Function1/3(aie)
  statek1/1 -> Bus Selector4/1
  Demux7/1 -> MATLAB Function/19(xl)
  Demux7/2 -> MATLAB Function/20(yl)
  Demux7/3 -> MATLAB Function/21(zl)
  Bus Selector4/1 -> Demux15/1, Demux7/1  "<xyz>"
  Demux14/1 -> MATLAB Function/22(vxl)
  Demux14/2 -> MATLAB Function/23(vyl)
  Demux14/3 -> MATLAB Function/24(vzl)
  Bus Selector4/2 -> Demux16/1, Demux14/1  "<xyz_dot>"
  Demux15/1 -> MATLAB Function4/13(xl)
  Demux15/2 -> MATLAB Function4/14(yl)
  Demux15/3 -> MATLAB Function4/15(zl)
  Demux16/1 -> MATLAB Function4/16(vxl)
  Demux16/2 -> MATLAB Function4/17(vyl)
  Demux16/3 -> MATLAB Function4/18(vzl)

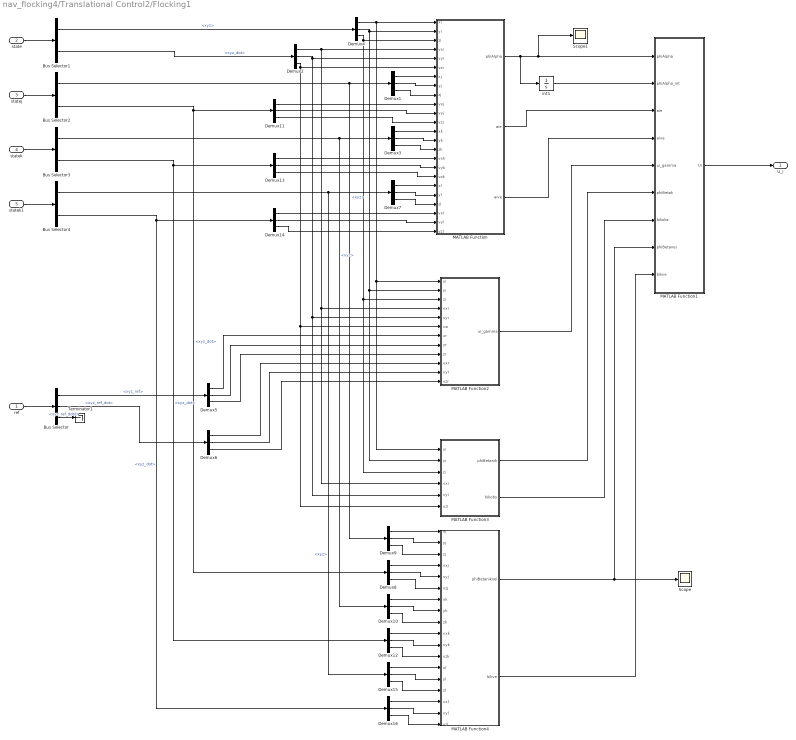
== system nav_flocking4/Translational Control2/Flocking1 ==
  ref : Inport
  state : Inport  Port=2
  statej : Inport  Port=3
  statek : Inport  Port=4
  statek1 : Inport  Port=5
  Bus Selector : BusSelector  OutputSignals=xyz_ref,xyz_ref_dot,xyz_ref_ddot
  Bus Selector{1..4} (4 alike) : BusSelector  OutputSignals=xyz,xyz_dot
  Demux{1..16} (16 alike) : Demux  Outputs=3
  MATLAB Function : MATLAB Function  TreatAsAtomicUnit=on
  MATLAB Function1 : MATLAB Function  TreatAsAtomicUnit=on
  MATLAB Function2 : MATLAB Function  TreatAsAtomicUnit=on
  MATLAB Function3 : MATLAB Function  TreatAsAtomicUnit=on
  MATLAB Function4 : MATLAB Function  TreatAsAtomicUnit=on
  Scope : Scope
  Scope1 : Scope
  Terminator1 : Terminator
  int1 : Integrator
  U_i : Outport  VectorParamsAs1DForOutWhenUnconnected=off
  wires:
  ref/1 -> Bus Selector/1
  state/1 -> Bus Selector1/1
  Bus Selector/2 -> Demux6/1  "<xyz_ref_dot>"
  Bus Selector/1 -> Demux5/1  "<xyz_ref>"
  Bus Selector1/1 -> Demux4/1  "<xyz>"
  Demux6/1 -> MATLAB Function2/10(vxr)
  Demux6/2 -> MATLAB Function2/11(vyr)
  statej/1 -> Bus Selector2/1
  Bus Selector2/1 -> Demux9/1, Demux1/1  "<xyz>"
  Demux4/1 -> MATLAB Function3/1(xi), MATLAB Function2/1(xi), MATLAB Function/1(xi)
  Demux4/2 -> MATLAB Function3/2(yi), MATLAB Function2/2(yi), MATLAB Function/2(yi)
  Demux1/1 -> MATLAB Function/7(xj)
  Demux1/2 -> MATLAB Function/8(yj)
  Bus Selector2/2 -> Demux8/1, Demux11/1  "<xyz_dot>"
  int1/1 -> MATLAB Function1/2(phiAlpha_int)
  MATLAB Function2/1(ui_gamma) -> MATLAB Function1/5(ui_gamma)
  statek/1 -> Bus Selector3/1
  Bus Selector3/2 -> Demux12/1, Demux13/1  "<xyz_dot>"
  Demux3/1 -> MATLAB Function/13(xk)
  Demux3/2 -> MATLAB Function/14(yk)
  Bus Selector3/1 -> Demux10/1, Demux3/1  "<xyz>"
  Demux9/1 -> MATLAB Function4/1(xj)
  Demux9/2 -> MATLAB Function4/2(yj)
  Demux10/1 -> MATLAB Function4/7(xk)
  Demux10/2 -> MATLAB Function4/8(yk)
  MATLAB Function/1(phiAlpha) -> int1/1, Scope1/1, MATLAB Function1/1(phiAlpha)
  Demux5/1 -> MATLAB Function2/7(xr)
  Demux5/2 -> MATLAB Function2/8(yr)
  Bus Selector1/2 -> Demux2/1  "<xyz_dot>"
  Demux4/3 -> MATLAB Function3/3(zi), MATLAB Function2/3(zi), MATLAB Function/3(zi)
  Demux3/3 -> MATLAB Function/15(zk)
  Demux5/3 -> MATLAB Function2/9(zr)
  Demux6/3 -> MATLAB Function2/12(vzr)
  MATLAB Function1/1(Ui) -> U_i/1
  Demux2/1 -> MATLAB Function2/4(vxi), MATLAB Function3/4(vxi), MATLAB Function/4(vxi)
  Demux2/2 -> MATLAB Function3/5(vyi), MATLAB Function2/5(vyi), MATLAB Function/5(vyi)
  Demux2/3 -> MATLAB Function3/6(vzi), MATLAB Function2/6(vzi), MATLAB Function/6(vzi)
  Demux1/3 -> MATLAB Function/9(zj)
  Demux11/1 -> MATLAB Function/10(vxj)
  Demux11/2 -> MATLAB Function/11(vyj)
  Demux11/3 -> MATLAB Function/12(vzj)
  Demux13/1 -> MATLAB Function/16(vxk)
  Demux13/2 -> MATLAB Function/17(vyk)
  Demux13/3 -> MATLAB Function/18(vzk)
  MATLAB Function/3(aive) -> MATLAB Function1/4(aive)
  Demux9/3 -> MATLAB Function4/3(zj)
  Demux10/3 -> MATLAB Function4/9(zk)
  MATLAB Function4/1(phiBetaniknei) -> Scope/1, MATLAB Function1/8(phiBetanei)
  Bus Selector/3 -> Terminator1/1  "<xyz_ref_ddot>"
  Demux8/1 -> MATLAB Function4/4(vxj)
  Demux8/2 -> MATLAB Function4/5(vyj)
  Demux8/3 -> MATLAB Function4/6(vzj)
  Demux12/1 -> MATLAB Function4/10(vxk)
  Demux12/2 -> MATLAB Function4/11(vyk)
  Demux12/3 -> MATLAB Function4/12(vzk)
  MATLAB Function4/2(bikve) -> MATLAB Function1/9(bikve)
  MATLAB Function3/1(phiBetanik) -> MATLAB Function1/6(phiBetak)
  MATLAB Function3/2(bikobs) -> MATLAB Function1/7(bikobs)
  MATLAB Function/2(aie) -> MATLAB Function1/3(aie)
  statek1/1 -> Bus Selector4/1
  Demux7/1 -> MATLAB Function/19(xl)
  Demux7/2 -> MATLAB Function/20(yl)
  Demux7/3 -> MATLAB Function/21(zl)
  Bus Selector4/1 -> Demux15/1, Demux7/1  "<xyz>"
  Demux14/1 -> MATLAB Function/22(vxl)
  Demux14/2 -> MATLAB Function/23(vyl)
  Demux14/3 -> MATLAB Function/24(vzl)
  Bus Selector4/2 -> Demux16/1, Demux14/1  "<xyz_dot>"
  Demux15/1 -> MATLAB Function4/13(xl)
  Demux15/2 -> MATLAB Function4/14(yl)
  Demux15/3 -> MATLAB Function4/15(zl)
  Demux16/1 -> MATLAB Function4/16(vxl)
  Demux16/2 -> MATLAB Function4/17(vyl)
  Demux16/3 -> MATLAB Function4/18(vzl)

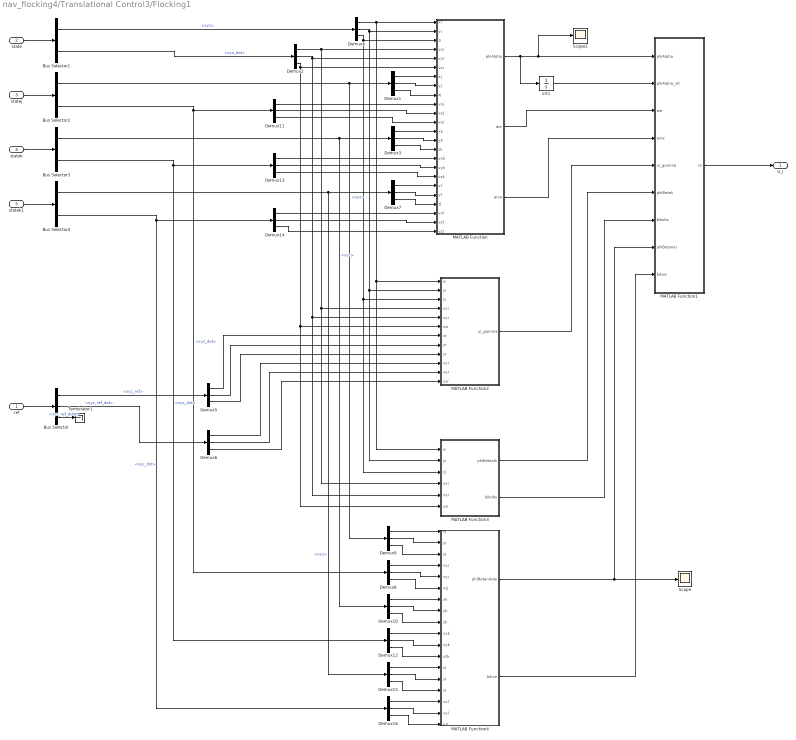
== system nav_flocking4/Translational Control3/Flocking1 ==
  ref : Inport
  state : Inport  Port=2
  statej : Inport  Port=3
  statek : Inport  Port=4
  statek1 : Inport  Port=5
  Bus Selector : BusSelector  OutputSignals=xyz_ref,xyz_ref_dot,xyz_ref_ddot
  Bus Selector{1..4} (4 alike) : BusSelector  OutputSignals=xyz,xyz_dot
  Demux{1..16} (16 alike) : Demux  Outputs=3
  MATLAB Function : MATLAB Function  TreatAsAtomicUnit=on
  MATLAB Function1 : MATLAB Function  TreatAsAtomicUnit=on
  MATLAB Function2 : MATLAB Function  TreatAsAtomicUnit=on
  MATLAB Function3 : MATLAB Function  TreatAsAtomicUnit=on
  MATLAB Function4 : MATLAB Function  TreatAsAtomicUnit=on
  Scope : Scope
  Scope1 : Scope
  Terminator1 : Terminator
  int1 : Integrator
  U_i : Outport  VectorParamsAs1DForOutWhenUnconnected=off
  wires:
  ref/1 -> Bus Selector/1
  state/1 -> Bus Selector1/1
  Bus Selector/2 -> Demux6/1  "<xyz_ref_dot>"
  Bus Selector/1 -> Demux5/1  "<xyz_ref>"
  Bus Selector1/1 -> Demux4/1  "<xyz>"
  Demux6/1 -> MATLAB Function2/10(vxr)
  Demux6/2 -> MATLAB Function2/11(vyr)
  statej/1 -> Bus Selector2/1
  Bus Selector2/1 -> Demux9/1, Demux1/1  "<xyz>"
  Demux4/1 -> MATLAB Function3/1(xi), MATLAB Function2/1(xi), MATLAB Function/1(xi)
  Demux4/2 -> MATLAB Function3/2(yi), MATLAB Function2/2(yi), MATLAB Function/2(yi)
  Demux1/1 -> MATLAB Function/7(xj)
  Demux1/2 -> MATLAB Function/8(yj)
  Bus Selector2/2 -> Demux8/1, Demux11/1  "<xyz_dot>"
  int1/1 -> MATLAB Function1/2(phiAlpha_int)
  MATLAB Function2/1(ui_gamma) -> MATLAB Function1/5(ui_gamma)
  statek/1 -> Bus Selector3/1
  Bus Selector3/2 -> Demux12/1, Demux13/1  "<xyz_dot>"
  Demux3/1 -> MATLAB Function/13(xk)
  Demux3/2 -> MATLAB Function/14(yk)
  Bus Selector3/1 -> Demux10/1, Demux3/1  "<xyz>"
  Demux9/1 -> MATLAB Function4/1(xj)
  Demux9/2 -> MATLAB Function4/2(yj)
  Demux10/1 -> MATLAB Function4/7(xk)
  Demux10/2 -> MATLAB Function4/8(yk)
  MATLAB Function/1(phiAlpha) -> int1/1, Scope1/1, MATLAB Function1/1(phiAlpha)
  Demux5/1 -> MATLAB Function2/7(xr)
  Demux5/2 -> MATLAB Function2/8(yr)
  Bus Selector1/2 -> Demux2/1  "<xyz_dot>"
  Demux4/3 -> MATLAB Function3/3(zi), MATLAB Function2/3(zi), MATLAB Function/3(zi)
  Demux3/3 -> MATLAB Function/15(zk)
  Demux5/3 -> MATLAB Function2/9(zr)
  Demux6/3 -> MATLAB Function2/12(vzr)
  MATLAB Function1/1(Ui) -> U_i/1
  Demux2/1 -> MATLAB Function2/4(vxi), MATLAB Function3/4(vxi), MATLAB Function/4(vxi)
  Demux2/2 -> MATLAB Function3/5(vyi), MATLAB Function2/5(vyi), MATLAB Function/5(vyi)
  Demux2/3 -> MATLAB Function3/6(vzi), MATLAB Function2/6(vzi), MATLAB Function/6(vzi)
  Demux1/3 -> MATLAB Function/9(zj)
  Demux11/1 -> MATLAB Function/10(vxj)
  Demux11/2 -> MATLAB Function/11(vyj)
  Demux11/3 -> MATLAB Function/12(vzj)
  Demux13/1 -> MATLAB Function/16(vxk)
  Demux13/2 -> MATLAB Function/17(vyk)
  Demux13/3 -> MATLAB Function/18(vzk)
  MATLAB Function/3(aive) -> MATLAB Function1/4(aive)
  Demux9/3 -> MATLAB Function4/3(zj)
  Demux10/3 -> MATLAB Function4/9(zk)
  MATLAB Function4/1(phiBetaniknei) -> Scope/1, MATLAB Function1/8(phiBetanei)
  Bus Selector/3 -> Terminator1/1  "<xyz_ref_ddot>"
  Demux8/1 -> MATLAB Function4/4(vxj)
  Demux8/2 -> MATLAB Function4/5(vyj)
  Demux8/3 -> MATLAB Function4/6(vzj)
  Demux12/1 -> MATLAB Function4/10(vxk)
  Demux12/2 -> MATLAB Function4/11(vyk)
  Demux12/3 -> MATLAB Function4/12(vzk)
  MATLAB Function4/2(bikve) -> MATLAB Function1/9(bikve)
  MATLAB Function3/1(phiBetanik) -> MATLAB Function1/6(phiBetak)
  MATLAB Function3/2(bikobs) -> MATLAB Function1/7(bikobs)
  MATLAB Function/2(aie) -> MATLAB Function1/3(aie)
  statek1/1 -> Bus Selector4/1
  Demux7/1 -> MATLAB Function/19(xl)
  Demux7/2 -> MATLAB Function/20(yl)
  Demux7/3 -> MATLAB Function/21(zl)
  Bus Selector4/1 -> Demux15/1, Demux7/1  "<xyz>"
  Demux14/1 -> MATLAB Function/22(vxl)
  Demux14/2 -> MATLAB Function/23(vyl)
  Demux14/3 -> MATLAB Function/24(vzl)
  Bus Selector4/2 -> Demux16/1, Demux14/1  "<xyz_dot>"
  Demux15/1 -> MATLAB Function4/13(xl)
  Demux15/2 -> MATLAB Function4/14(yl)
  Demux15/3 -> MATLAB Function4/15(zl)
  Demux16/1 -> MATLAB Function4/16(vxl)
  Demux16/2 -> MATLAB Function4/17(vyl)
  Demux16/3 -> MATLAB Function4/18(vzl)

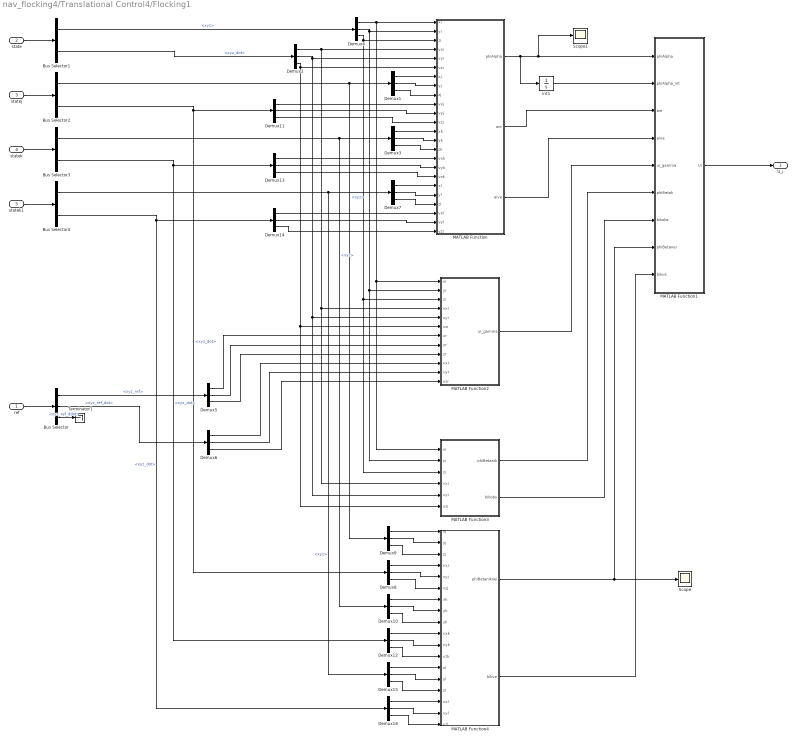
== system nav_flocking4/Translational Control4/Flocking1 ==
  ref : Inport
  state : Inport  Port=2
  statej : Inport  Port=3
  statek : Inport  Port=4
  statek1 : Inport  Port=5
  Bus Selector : BusSelector  OutputSignals=xyz_ref,xyz_ref_dot,xyz_ref_ddot
  Bus Selector{1..4} (4 alike) : BusSelector  OutputSignals=xyz,xyz_dot
  Demux{1..16} (16 alike) : Demux  Outputs=3
  MATLAB Function : MATLAB Function  TreatAsAtomicUnit=on
  MATLAB Function1 : MATLAB Function  TreatAsAtomicUnit=on
  MATLAB Function2 : MATLAB Function  TreatAsAtomicUnit=on
  MATLAB Function3 : MATLAB Function  TreatAsAtomicUnit=on
  MATLAB Function4 : MATLAB Function  TreatAsAtomicUnit=on
  Scope : Scope
  Scope1 : Scope
  Terminator1 : Terminator
  int1 : Integrator
  U_i : Outport  VectorParamsAs1DForOutWhenUnconnected=off
  wires:
  ref/1 -> Bus Selector/1
  state/1 -> Bus Selector1/1
  Bus Selector/2 -> Demux6/1  "<xyz_ref_dot>"
  Bus Selector/1 -> Demux5/1  "<xyz_ref>"
  Bus Selector1/1 -> Demux4/1  "<xyz>"
  Demux6/1 -> MATLAB Function2/10(vxr)
  Demux6/2 -> MATLAB Function2/11(vyr)
  statej/1 -> Bus Selector2/1
  Bus Selector2/1 -> Demux9/1, Demux1/1  "<xyz>"
  Demux4/1 -> MATLAB Function3/1(xi), MATLAB Function2/1(xi), MATLAB Function/1(xi)
  Demux4/2 -> MATLAB Function3/2(yi), MATLAB Function2/2(yi), MATLAB Function/2(yi)
  Demux1/1 -> MATLAB Function/7(xj)
  Demux1/2 -> MATLAB Function/8(yj)
  Bus Selector2/2 -> Demux8/1, Demux11/1  "<xyz_dot>"
  int1/1 -> MATLAB Function1/2(phiAlpha_int)
  MATLAB Function2/1(ui_gamma) -> MATLAB Function1/5(ui_gamma)
  statek/1 -> Bus Selector3/1
  Bus Selector3/2 -> Demux12/1, Demux13/1  "<xyz_dot>"
  Demux3/1 -> MATLAB Function/13(xk)
  Demux3/2 -> MATLAB Function/14(yk)
  Bus Selector3/1 -> Demux10/1, Demux3/1  "<xyz>"
  Demux9/1 -> MATLAB Function4/1(xj)
  Demux9/2 -> MATLAB Function4/2(yj)
  Demux10/1 -> MATLAB Function4/7(xk)
  Demux10/2 -> MATLAB Function4/8(yk)
  MATLAB Function/1(phiAlpha) -> int1/1, Scope1/1, MATLAB Function1/1(phiAlpha)
  Demux5/1 -> MATLAB Function2/7(xr)
  Demux5/2 -> MATLAB Function2/8(yr)
  Bus Selector1/2 -> Demux2/1  "<xyz_dot>"
  Demux4/3 -> MATLAB Function3/3(zi), MATLAB Function2/3(zi), MATLAB Function/3(zi)
  Demux3/3 -> MATLAB Function/15(zk)
  Demux5/3 -> MATLAB Function2/9(zr)
  Demux6/3 -> MATLAB Function2/12(vzr)
  MATLAB Function1/1(Ui) -> U_i/1
  Demux2/1 -> MATLAB Function2/4(vxi), MATLAB Function3/4(vxi), MATLAB Function/4(vxi)
  Demux2/2 -> MATLAB Function3/5(vyi), MATLAB Function2/5(vyi), MATLAB Function/5(vyi)
  Demux2/3 -> MATLAB Function3/6(vzi), MATLAB Function2/6(vzi), MATLAB Function/6(vzi)
  Demux1/3 -> MATLAB Function/9(zj)
  Demux11/1 -> MATLAB Function/10(vxj)
  Demux11/2 -> MATLAB Function/11(vyj)
  Demux11/3 -> MATLAB Function/12(vzj)
  Demux13/1 -> MATLAB Function/16(vxk)
  Demux13/2 -> MATLAB Function/17(vyk)
  Demux13/3 -> MATLAB Function/18(vzk)
  MATLAB Function/3(aive) -> MATLAB Function1/4(aive)
  Demux9/3 -> MATLAB Function4/3(zj)
  Demux10/3 -> MATLAB Function4/9(zk)
  MATLAB Function4/1(phiBetaniknei) -> Scope/1, MATLAB Function1/8(phiBetanei)
  Bus Selector/3 -> Terminator1/1  "<xyz_ref_ddot>"
  Demux8/1 -> MATLAB Function4/4(vxj)
  Demux8/2 -> MATLAB Function4/5(vyj)
  Demux8/3 -> MATLAB Function4/6(vzj)
  Demux12/1 -> MATLAB Function4/10(vxk)
  Demux12/2 -> MATLAB Function4/11(vyk)
  Demux12/3 -> MATLAB Function4/12(vzk)
  MATLAB Function4/2(bikve) -> MATLAB Function1/9(bikve)
  MATLAB Function3/1(phiBetanik) -> MATLAB Function1/6(phiBetak)
  MATLAB Function3/2(bikobs) -> MATLAB Function1/7(bikobs)
  MATLAB Function/2(aie) -> MATLAB Function1/3(aie)
  statek1/1 -> Bus Selector4/1
  Demux7/1 -> MATLAB Function/19(xl)
  Demux7/2 -> MATLAB Function/20(yl)
  Demux7/3 -> MATLAB Function/21(zl)
  Bus Selector4/1 -> Demux15/1, Demux7/1  "<xyz>"
  Demux14/1 -> MATLAB Function/22(vxl)
  Demux14/2 -> MATLAB Function/23(vyl)
  Demux14/3 -> MATLAB Function/24(vzl)
  Bus Selector4/2 -> Demux16/1, Demux14/1  "<xyz_dot>"
  Demux15/1 -> MATLAB Function4/13(xl)
  Demux15/2 -> MATLAB Function4/14(yl)
  Demux15/3 -> MATLAB Function4/15(zl)
  Demux16/1 -> MATLAB Function4/16(vxl)
  Demux16/2 -> MATLAB Function4/17(vyl)
  Demux16/3 -> MATLAB Function4/18(vzl)
